simulink model "UnlinearSimulation2ArmOnly"  (R2017a)
settings: Solver=VariableStepAuto  StartTime=0.0  StopTime=5  RelTol=1e-3
libraries: simulink x1
settings Model: Creator=khrom  LastModifiedBy=khrom

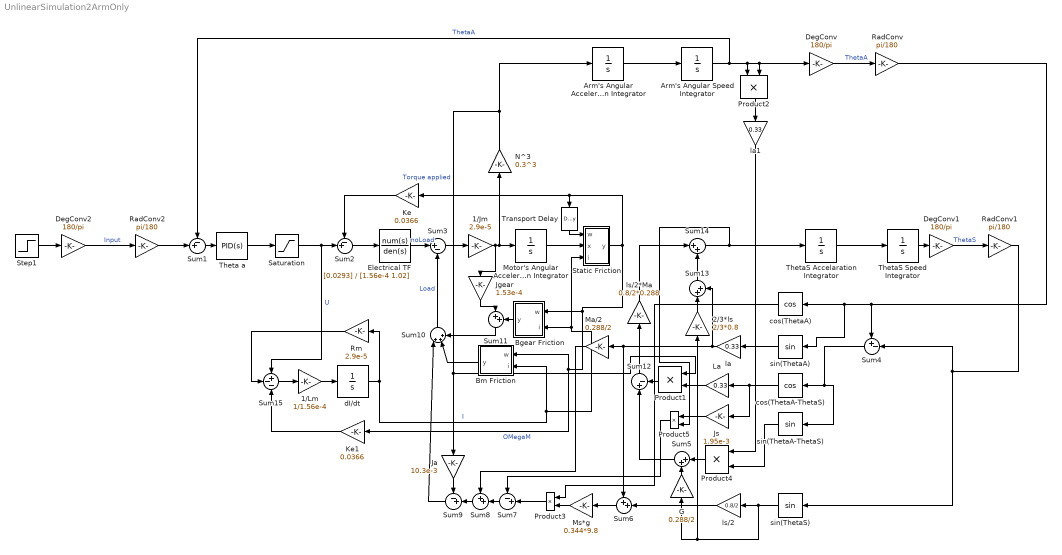
== system UnlinearSimulation2ArmOnly ==
  1/Jm : Gain  Gain=2.9e-5
  1/Lm : Gain  Gain=1/1.56e-4
  2/3*ls : Gain  Gain=2/3*0.8
  Arm's Angular Acceleration Integrator : TransferFcn  Denominator=[1 0]
  Arm's Angular Speed Integrator : TransferFcn  Denominator=[1 0]
  Bgear Friction : MATLAB Function  TreatAsAtomicUnit=on
  Bm Friction : MATLAB Function  TreatAsAtomicUnit=on
  DegConv : Gain  Gain=180/pi
  DegConv1 : Gain  Gain=180/pi
  DegConv2 : Gain  Gain=180/pi
  Electrical TF : TransferFcn  Numerator=[0.0293]  Denominator=[1.56e-4 1.02]
  G : Gain  Gain=0.288/2
  Ja : Gain  Gain=10.3e-3
  Jgear : Gain  Gain=1.53e-4
  Js : Gain  Gain=1.95e-3
  Ke : Gain  Gain=0.0366
  Ke1 : Gain  Gain=0.0366
  La : Gain  Gain=0.33
  Ma/2 : Gain  Gain=0.288/2
  Motor's Angular Acceleration Integrator : TransferFcn  Denominator=[1 0]
  Ms*g : Gain  Gain=0.344*9.8
  N^3 : Gain  Gain=0.3^3
  Product{1..5} (5 alike) : Product
  RadConv : Gain  Gain=pi/180
  RadConv1 : Gain  Gain=pi/180
  RadConv2 : Gain  Gain=pi/180
  Rm : Gain  Gain=2.9e-5
  Saturation : Saturate  UpperLimit=14  LowerLimit=-14
  Static Friction : MATLAB Function  TreatAsAtomicUnit=on
  Step1 : Step  Time=0  After=5*pi/180  SampleTime=0
  Sum{1..2,7,9} (4 alike) : Sum  Inputs=-+|
  Sum10 : Sum  Inputs=|+++
  Sum{5,11,13..14} (4 alike) : Sum  Inputs=|++
  Sum12 : Sum  Inputs=|+-
  Sum15 : Sum  Inputs=+--
  Sum3 : Sum  Inputs=|+-
  Sum4 : Sum  Inputs=+-|
  Sum6 : Sum  Inputs=++|
  Sum8 : Sum  Inputs=++|
  Theta a : simulink/Continuous/PID Controller  Controller=PID  TimeDomain=Continuous-time  SampleTime=-1  IntegratorMethod=Forward Euler  FilterMethod=Forward Euler  Form=Parallel  UseFilter=on  ControllerParametersSource=internal  P=400  I=900  D=25  N=100  InitialConditionSource=internal  InitialConditionForIntegrator=0  InitialConditionForFilter=0  ExternalReset=none  LimitOutput=off  UpperSaturationLimit=inf  LowerSaturationLimit=-inf  LinearizeAsGain=on  AntiWindupMode=none  Kb=1  TrackingMode=off  Kt=1  PParamMin=[]  PParamMax=[]  IParamMin=[]  IParamMax=[]  DParamMin=[]  DParamMax=[]  NParamMin=[]  NParamMax=[]  KbParamMin=[]  KbParamMax=[]  KtParamMin=[]  KtParamMax=[]  POutMin=[]  POutMax=[]  IOutMin=[]  IOutMax=[]  DOutMin=[]  DOutMax=[]  NOutMin=[]  NOutMax=[]  KbOutMin=[]  KbOutMax=[]  KtOutMin=[]  KtOutMax=[]  IntegratorOutMin=[]  IntegratorOutMax=[]  FilterOutMin=[]  FilterOutMax=[]  SumOutMin=[]  SumOutMax=[]  SumI1OutMin=[]  SumI1OutMax=[]  SumI2OutMin=[]  SumI2OutMax=[]  SumI3OutMin=[]  SumI3OutMax=[]  SumDOutMin=[]  SumDOutMax=[]  SaturationOutMin=[]  SaturationOutMax=[]  IntegratorContinuousStateAttributes=''  IntegratorStateMustResolveToSignalObject=off  IntegratorRTWStateStorageClass=Auto  FilterContinuousStateAttributes=''  FilterStateMustResolveToSignalObject=off  FilterRTWStateStorageClass=Auto  DifferentiatorICPrevScaledInput=0  DifferentiatorOutMin=[]  DifferentiatorOutMax=[]  InitialConditionSetting=State (most efficient)
  ThetaS Accelaration Integrator : TransferFcn  Denominator=[1 0]
  ThetaS Speed Integrator : TransferFcn  Denominator=[1 0]
  Transport Delay : TransportDelay  DelayTime=0.000000000000000000000000001
  cos(ThetaA) : Trigonometry  Operator=cos
  cos(ThetaA-ThetaS) : Trigonometry  Operator=cos
  dI/dt : TransferFcn  Denominator=[1 0]
  la : Gain  Gain=0.33
  la1 : Gain  Gain=0.33
  ls/2 : Gain  Gain=0.8/2
  ls/2*Ma : Gain  Gain=0.8/2*0.288
  sin(ThetaA) : Trigonometry
  sin(ThetaA-ThetaS) : Trigonometry
  sin(ThetaS) : Trigonometry
  wires:
  Sum1/1 -> Theta a/1
  ThetaS Accelaration Integrator/1 -> ThetaS Speed Integrator/1
  Arm's Angular Acceleration Integrator/1 -> Arm's Angular Speed Integrator/1
  Theta a/1 -> Saturation/1
  Sum3/1 -> 1/Jm/1
  Sum2/1 -> Electrical TF/1
  Static Friction/1(y) -> Ke1/1, Bm Friction/1(w), Bgear Friction/1(w), Ke/1, Transport Delay/1  "OMegaM"
  Ke/1 -> Sum2/1
  Electrical TF/1 -> Sum3/1  "noLoad"
  1/Jm/1 -> Motor's Angular Acceleration Integrator/1, N^3/1, Jgear/1
  Arm's Angular Speed Integrator/1 -> Sum1/1, Product2/1, Product2/2, DegConv/1  "ThetaA"
  ThetaS Speed Integrator/1 -> DegConv1/1
  Sum4/1 -> sin(ThetaA-ThetaS)/1, cos(ThetaA-ThetaS)/1
  cos(ThetaA-ThetaS)/1 -> La/1, Js/1
  N^3/1 -> Product1/1, Ja/1, Arm's Angular Acceleration Integrator/1  "Torque applied"
  sin(ThetaA)/1 -> la/1
  sin(ThetaS)/1 -> 2/3*ls/1, G/1, ls/2/1
  ls/2/1 -> Sum6/2
  la/1 -> Sum13/2, Ma/2/1, Sum6/1
  Sum6/1 -> Ms*g/1
  Ms*g/1 -> Product3/2
  cos(ThetaA)/1 -> Product3/1
  Product3/1 -> Sum7/2
  Js/1 -> Product5/1
  Ma/2/1 -> Sum8/1
  Sum7/1 -> Sum8/2
  Sum8/1 -> Sum9/2
  Ja/1 -> Sum9/1
  Sum9/1 -> Sum10/1
  Sum10/1 -> Sum3/2  "Load"
  Jgear/1 -> Sum11/1
  Sum11/1 -> Sum10/3
  La/1 -> Product1/2
  Product2/1 -> la1/1
  sin(ThetaA-ThetaS)/1 -> Product4/2
  la1/1 -> Product4/1
  G/1 -> Sum5/2
  Product4/1 -> Sum5/1
  Product1/1 -> Sum12/2
  Sum5/1 -> Sum12/1
  Sum12/1 -> ls/2*Ma/1
  Sum14/1 -> Product5/2, ThetaS Accelaration Integrator/1
  2/3*ls/1 -> Sum13/1
  Sum13/1 -> Sum14/2
  ls/2*Ma/1 -> Sum14/1
  Step1/1 -> DegConv2/1
  Bm Friction/1(y) -> Sum10/2
  dI/dt/1 -> Static Friction/3(i), Bgear Friction/2(i), Bm Friction/2(i), Rm/1  "I"
  Sum15/1 -> 1/Lm/1
  Rm/1 -> Sum15/2
  Ke1/1 -> Sum15/3
  Motor's Angular Acceleration Integrator/1 -> Static Friction/2(x)
  Transport Delay/1 -> Static Friction/1(w)
  Bgear Friction/1(y) -> Sum11/2
  Saturation/1 -> Sum15/1, Sum2/2  "U"
  DegConv/1 -> RadConv/1  "ThetaA"
  RadConv/1 -> Sum4/1, sin(ThetaA)/1, cos(ThetaA)/1
  DegConv1/1 -> RadConv1/1  "ThetaS"
  RadConv1/1 -> sin(ThetaS)/1, Sum4/2
  Product5/1 -> Sum7/1
  1/Lm/1 -> dI/dt/1
  DegConv2/1 -> RadConv2/1  "Input"
  RadConv2/1 -> Sum1/2

== matlab function UnlinearSimulation2ArmOnly/Bm Friction ==
  data: w input; y output; i input
function y = fcn(w,i)

Bm=1.59e-4;
imini=0.64;
Kt=0.0293;

if w~=0
    y=Bm*w;
elseif abs(i)>imini
    y=Kt*imini;
else
    y=Kt*i;
end

== matlab function UnlinearSimulation2ArmOnly/Static Friction ==
  data: w input; x input; y output; i input
function y = fcn(w,x,i)

Bm=1.59e-4;
imini=1.35;

if w~=0
    y=x;
elseif abs(i)>imini
    y=x;
else
    y=0;
end

== matlab function UnlinearSimulation2ArmOnly/Bgear Friction ==
  data: w input; y output; i input
function y = fcn(w,i)

Bgear=1.11e-3;
imini=1.35;
Kt=0.0293;
N=0.3;

if w~=0
    y=Bgear*w;
elseif abs(i)>imini
    y=Kt*imini/N^3;
else
    y=Kt*i/N^3;
end
